simulink model "es01_sim"  (R2021b)
settings: Solver=VariableStepAuto  StartTime=0.0  StopTime=10000  RelTol=1e-3
undefined symbols (not defined in the file): m
libraries: simulink x8
settings Model: Creator=francescafornasier  LastModifiedBy=francescafornasier

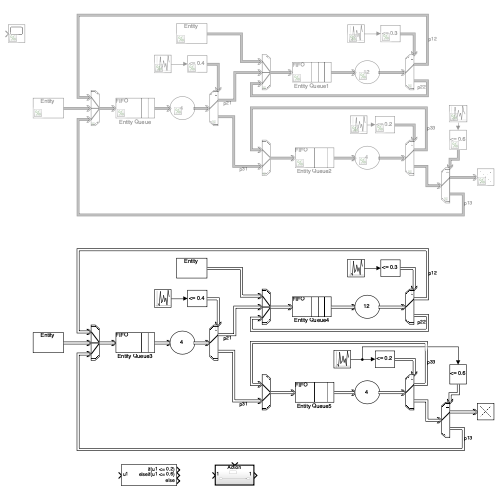
[thumbnail: Simulink's stored preview of the top-level diagram]
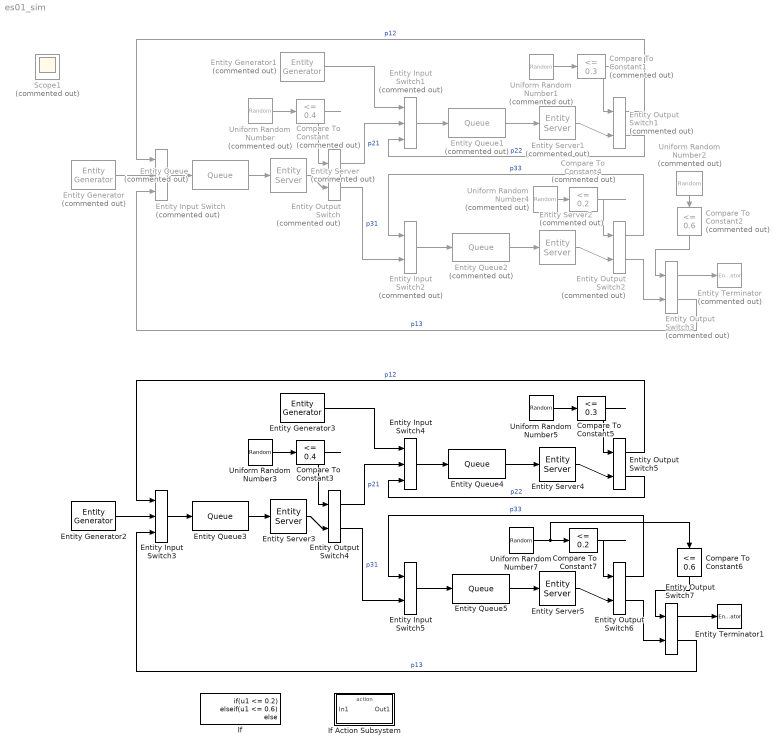
== system es01_sim ==
  Compare To Constant : simulink/Logic and Bit Operations/Compare To Constant  Commented=on  relop=<=  const=0.4  OutDataTypeStr=boolean
  Compare To Constant1 : simulink/Logic and Bit Operations/Compare To Constant  Commented=on  relop=<=  const=0.3  OutDataTypeStr=boolean
  Compare To Constant2 : simulink/Logic and Bit Operations/Compare To Constant  Commented=on  relop=<=  const=0.6  OutDataTypeStr=boolean
  Compare To Constant3 : simulink/Logic and Bit Operations/Compare To Constant  relop=<=  const=0.4  OutDataTypeStr=boolean
  Compare To Constant4 : simulink/Logic and Bit Operations/Compare To Constant  Commented=on  relop=<=  const=0.2  OutDataTypeStr=boolean
  Compare To Constant5 : simulink/Logic and Bit Operations/Compare To Constant  relop=<=  const=0.3  OutDataTypeStr=boolean
  Compare To Constant6 : simulink/Logic and Bit Operations/Compare To Constant  relop=<=  const=0.6  OutDataTypeStr=boolean
  Compare To Constant7 : simulink/Logic and Bit Operations/Compare To Constant  relop=<=  const=0.2  OutDataTypeStr=boolean
  Entity Input Switch : EntityInputSwitch  Commented=on  InputPortMessageModes=m,m,m  OutputPortMessageModes=m  NumberInputPorts=3
      settings: InputPortMap=u1,u2,u3
  Entity Input Switch1 : EntityInputSwitch  Commented=on  InputPortMessageModes=m,m,m  OutputPortMessageModes=m  NumberInputPorts=3
      settings: InputPortMap=u1,u2,u3
  Entity Input Switch2 : EntityInputSwitch  Commented=on  InputPortMessageModes=m,m  OutputPortMessageModes=m
  Entity Input Switch3 : EntityInputSwitch  InputPortMessageModes=m,m,m  OutputPortMessageModes=m  NumberInputPorts=3
      settings: InputPortMap=u1,u2,u3
  Entity Input Switch4 : EntityInputSwitch  InputPortMessageModes=m,m,m  OutputPortMessageModes=m  NumberInputPorts=3
      settings: InputPortMap=u1,u2,u3
  Entity Input Switch5 : EntityInputSwitch  InputPortMessageModes=m,m  OutputPortMessageModes=m
  Entity Output Switch{,1..3} (4 alike) : EntityOutputSwitch  Commented=on  InputPortMessageModes=m,m  OutputPortMessageModes=m,m  SwitchingCriterion=From control port  SwitchAttributeName=Attribute1
      settings: InputPortMap=u0,u1
  Entity Output Switch{4..7} (4 alike) : EntityOutputSwitch  InputPortMessageModes=m,m  OutputPortMessageModes=m,m  SwitchingCriterion=From control port  SwitchAttributeName=Attribute1
      settings: InputPortMap=u0,u1
  Entity Generator : EntityGenerator  Commented=on  OutputPortMessageModes=m  Period=2  EntityType=Structured  EntityTypeName=Entity
  Entity Generator1 : EntityGenerator  Commented=on  OutputPortMessageModes=m  Period=2  EntityType=Structured  EntityTypeName=Entity
  Entity Generator2 : EntityGenerator  OutputPortMessageModes=m  TimeSource=MATLAB action  Period=2  EntityType=Structured  EntityTypeName=Entity
  Entity Generator3 : EntityGenerator  OutputPortMessageModes=m  Period=2  EntityType=Structured  EntityTypeName=Entity
  Entity Queue : Queue  Commented=on  InputPortMessageModes=m  OutputPortMessageModes=m
  Entity Queue1 : Queue  Commented=on  InputPortMessageModes=m  OutputPortMessageModes=m
  Entity Queue2 : Queue  Commented=on  InputPortMessageModes=m  OutputPortMessageModes=m
  Entity Queue3 : Queue  InputPortMessageModes=m  OutputPortMessageModes=m
  Entity Queue4 : Queue  InputPortMessageModes=m  OutputPortMessageModes=m
  Entity Queue5 : Queue  InputPortMessageModes=m  OutputPortMessageModes=m
  Entity Server : EntityServer  Commented=on  InputPortMessageModes=m  OutputPortMessageModes=m  Capacity=4
  Entity Server1 : EntityServer  Commented=on  InputPortMessageModes=m  OutputPortMessageModes=m  Capacity=12
  Entity Server2 : EntityServer  Commented=on  InputPortMessageModes=m  OutputPortMessageModes=m  Capacity=4
  Entity Server3 : EntityServer  InputPortMessageModes=m  OutputPortMessageModes=m  Capacity=4
  Entity Server4 : EntityServer  InputPortMessageModes=m  OutputPortMessageModes=m  Capacity=12
  Entity Server5 : EntityServer  InputPortMessageModes=m  OutputPortMessageModes=m  Capacity=4
  Entity Terminator : EntityTerminator  Commented=on  InputPortMessageModes=m
  Entity Terminator1 : EntityTerminator  InputPortMessageModes=m
  If : If  IfExpression=u1 <= 0.2  ElseIfExpressions=u1 <= 0.6
  If Action Subsystem : Subsystem  TreatAsAtomicUnit=on
  Scope1 : Scope  Commented=on
  Uniform Random Number{,1..2,4} (4 alike) : UniformRandomNumber  Commented=on  Minimum=0  SampleTime=0.5
  Uniform Random Number3 : UniformRandomNumber  Minimum=0  SampleTime=0.5
  Uniform Random Number5 : UniformRandomNumber  Minimum=0  SampleTime=0.5
  Uniform Random Number7 : UniformRandomNumber  Minimum=0
  wires:
  Entity Queue/1 -> Entity Server/1
  Entity Input Switch/1 -> Entity Queue/1
  Entity Server/1 -> Entity Output Switch/2
  Entity Generator/1 -> Entity Input Switch/2
  Entity Output Switch/2 -> Entity Input Switch2/2  "p31"
  Entity Generator1/1 -> Entity Input Switch1/1
  Entity Input Switch1/1 -> Entity Queue1/1
  Entity Queue1/1 -> Entity Server1/1
  Entity Queue2/1 -> Entity Server2/1
  Entity Input Switch2/1 -> Entity Queue2/1
  Entity Server2/1 -> Entity Output Switch2/2
  Entity Server1/1 -> Entity Output Switch1/2
  Entity Output Switch/1 -> Entity Input Switch1/2  "p21"
  Entity Output Switch1/1 -> Entity Input Switch/1  "p12"
  Entity Output Switch1/2 -> Entity Input Switch1/3  "p22"
  Uniform Random Number/1 -> Compare To Constant/1
  Compare To Constant/1 -> Entity Output Switch/1
  Uniform Random Number1/1 -> Compare To Constant1/1
  Uniform Random Number2/1 -> Compare To Constant2/1
  Compare To Constant1/1 -> Entity Output Switch1/1
  Uniform Random Number4/1 -> Compare To Constant4/1
  Entity Output Switch2/2 -> Entity Output Switch3/2
  Entity Output Switch2/1 -> Entity Input Switch2/1  "p33"
  Compare To Constant4/1 -> Entity Output Switch2/1
  Compare To Constant2/1 -> Entity Output Switch3/1
  Entity Output Switch3/1 -> Entity Terminator/1
  Entity Output Switch3/2 -> Entity Input Switch/3  "p13"
  Entity Server5/1 -> Entity Output Switch6/2
  Entity Output Switch5/2 -> Entity Input Switch4/3  "p22"
  Entity Queue3/1 -> Entity Server3/1
  Compare To Constant5/1 -> Entity Output Switch5/1
  Entity Output Switch5/1 -> Entity Input Switch3/1  "p12"
  Entity Output Switch4/2 -> Entity Input Switch5/2  "p31"
  Entity Server4/1 -> Entity Output Switch5/2
  Entity Output Switch4/1 -> Entity Input Switch4/2  "p21"
  Entity Input Switch5/1 -> Entity Queue5/1
  Entity Output Switch7/1 -> Entity Terminator1/1
  Entity Input Switch4/1 -> Entity Queue4/1
  Entity Generator3/1 -> Entity Input Switch4/1
  Entity Input Switch3/1 -> Entity Queue3/1
  Entity Output Switch7/2 -> Entity Input Switch3/3  "p13"
  Entity Queue5/1 -> Entity Server5/1
  Compare To Constant3/1 -> Entity Output Switch4/1
  Uniform Random Number5/1 -> Compare To Constant5/1
  Compare To Constant7/1 -> Entity Output Switch6/1
  Uniform Random Number3/1 -> Compare To Constant3/1
  Entity Output Switch6/2 -> Entity Output Switch7/2
  Entity Server3/1 -> Entity Output Switch4/2
  Entity Queue4/1 -> Entity Server4/1
  Uniform Random Number7/1 -> Compare To Constant6/1, Compare To Constant7/1
  Compare To Constant6/1 -> Entity Output Switch7/1
  Entity Output Switch6/1 -> Entity Input Switch5/1  "p33"
  Entity Generator2/1 -> Entity Input Switch3/2

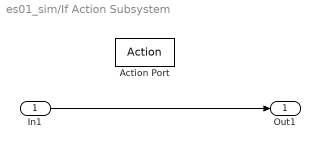
== system es01_sim/If Action Subsystem ==
  In1 : Inport
  Action Port : ActionPort
  Out1 : Outport
  wires:
  In1/1 -> Out1/1
